simulink model "VARIACION_P5"  (R2019b)
settings: Solver=VariableStepAuto  StartTime=0.0  StopTime=15000  RelTol=1e-3
undefined symbols (not defined in the file): n, p1, p2, p3, p6
libraries: simulink x10
settings Model: Creator=USUARIO  LastModifiedBy=USUARIO

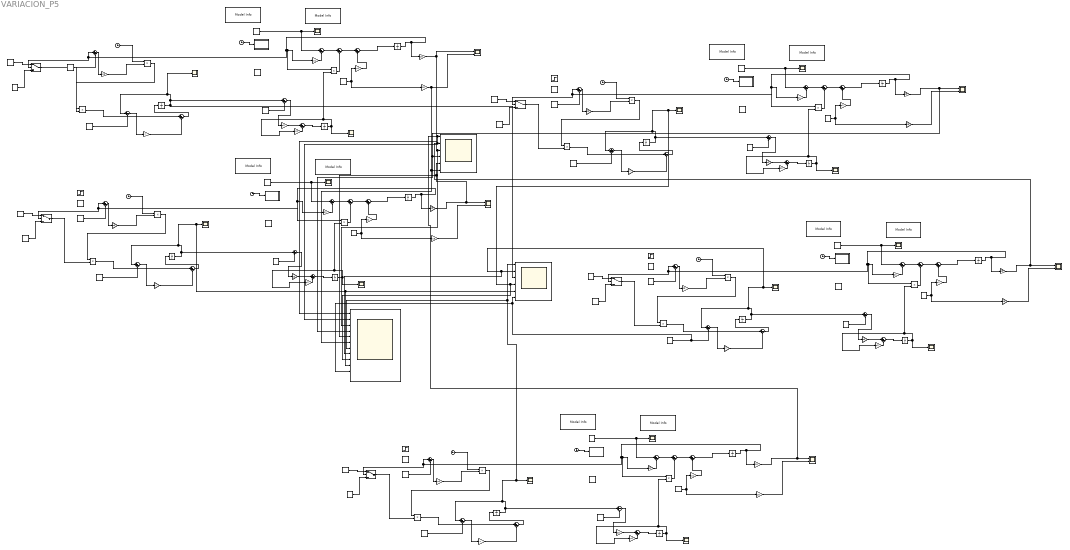
== system VARIACION_P5 ==
  Clock{,1..9} (10 alike) : Clock
  Constant{1..5} (5 alike) : Constant  Value=0
  Gain{1,5,7,11,13,17,19,23,25,29} (10 alike) : Gain  Gain=p1
  Gain{3..4,9..10,15..16,21..22,27..28} (10 alike) : Gain  Gain=18
  Gain{6,12,18,24,30} (5 alike) : Gain  Gain=p2
  Gain{2,8,14,20,26} (5 alike) : Gain  Gain=p3
  Glucosa {,1..3} (4 alike) : Constant  Value=7
  Glucosa basal{1..2,5,10,13} (5 alike) : Constant  Value=4.5
  Glucosa basal{3,6..7,11,14} (5 alike) : Constant
  Glucosa basal{4,8..9,12,15} (5 alike) : Constant  Value=0
  Grafica ingesta D{1..5} (5 alike) : Scope
  INSULINA{,1..4} (5 alike) : Scope
  Ib{,1..4} (5 alike) : Constant  Value=12
  Ingesta 75 g1 : MATLAB Function  TreatAsAtomicUnit=on
  Ingesta 75 g2 : MATLAB Function  TreatAsAtomicUnit=on
  Ingesta 75 g3 : MATLAB Function  TreatAsAtomicUnit=on
  Ingesta 75 g4 : MATLAB Function  TreatAsAtomicUnit=on
  Ingesta 75 g5 : MATLAB Function  TreatAsAtomicUnit=on
  Insulina basal{1..5} (5 alike) : Constant  Value=12
  Integrator{1,3,6,9,15} (5 alike) : Integrator  InitialCondition=7.5
  Integrator{4,7,10,12,14} (5 alike) : Integrator  InitialCondition=12
  Integrator{2,5,8,11,13} (5 alike) : Integrator
  Model Info1 : simulink/Model-Wide Utilities/Model Info  Frame=on  DisplayStringWithTags=|  HorizontalTextAlignment=Center  LeftAlignmentValue=0.5
      | Insulina constante 
      | igual a la basal
      | 
      | I(0) = Ib
  Model Info10 : simulink/Model-Wide Utilities/Model Info  Frame=on  DisplayStringWithTags=|  HorizontalTextAlignment=Center  LeftAlignmentValue=0.5
      | MODELO ORIGINAL
      | 
      | 
      | PERSONA NO DIABETICA
      | 
      | CON INSULINA VARIABLE
  Model Info2 : simulink/Model-Wide Utilities/Model Info  Frame=on  DisplayStringWithTags=|  HorizontalTextAlignment=Center  LeftAlignmentValue=0.5
      | MODELO ORIGINAL
      | 
      | 
      | PERSONA NO DIABETICA
      | 
      | CON INSULINA VARIABLE
  Model Info3 : simulink/Model-Wide Utilities/Model Info  Frame=on  DisplayStringWithTags=|  HorizontalTextAlignment=Center  LeftAlignmentValue=0.5
      | Insulina constante 
      | igual a la basal
      | 
      | I(0) = Ib
  Model Info4 : simulink/Model-Wide Utilities/Model Info  Frame=on  DisplayStringWithTags=|  HorizontalTextAlignment=Center  LeftAlignmentValue=0.5
      | MODELO ORIGINAL
      | 
      | 
      | PERSONA NO DIABETICA
      | 
      | CON INSULINA VARIABLE
  Model Info5 : simulink/Model-Wide Utilities/Model Info  Frame=on  DisplayStringWithTags=|  HorizontalTextAlignment=Center  LeftAlignmentValue=0.5
      | Insulina constante 
      | igual a la basal
      | 
      | I(0) = Ib
  Model Info6 : simulink/Model-Wide Utilities/Model Info  Frame=on  DisplayStringWithTags=|  HorizontalTextAlignment=Center  LeftAlignmentValue=0.5
      | MODELO ORIGINAL
      | 
      | 
      | PERSONA NO DIABETICA
      | 
      | CON INSULINA VARIABLE
  Model Info7 : simulink/Model-Wide Utilities/Model Info  Frame=on  DisplayStringWithTags=|  HorizontalTextAlignment=Center  LeftAlignmentValue=0.5
      | Insulina constante 
      | igual a la basal
      | 
      | I(0) = Ib
  Model Info8 : simulink/Model-Wide Utilities/Model Info  Frame=on  DisplayStringWithTags=|  HorizontalTextAlignment=Center  LeftAlignmentValue=0.5
      | MODELO ORIGINAL
      | 
      | 
      | PERSONA NO DIABETICA
      | 
      | CON INSULINA VARIABLE
  Model Info9 : simulink/Model-Wide Utilities/Model Info  Frame=on  DisplayStringWithTags=|  HorizontalTextAlignment=Center  LeftAlignmentValue=0.5
      | Insulina constante 
      | igual a la basal
      | 
      | I(0) = Ib
  Product{1..15} (15 alike) : Product
  Step{,1..3} (4 alike) : Step  Time=10  Before=7  After=4  SampleTime=0
  Sum{1..2,4..7,9..15,17..23,25..34,36..40} (35 alike) : Sum  Inputs=|+-
  Sum{3,8,16,24,35} (5 alike) : Sum  Inputs=|++
  Switch : Switch  Criteria=u2 > Threshold  Threshold=5
  Switch1 : Switch  Criteria=u2 > Threshold  Threshold=5.556
  Switch2 : Switch  Criteria=u2 > Threshold  Threshold=5.278
  Switch3 : Switch  Criteria=u2 > Threshold  Threshold=4.7222
  Switch4 : Switch  Criteria=u2 > Threshold  Threshold=4.5
  i(T){1..5} (5 alike) : Constant  Value=12
  insulina activa{1..5} (5 alike) : Scope
  mODELO ORIGINAL{1..5} (5 alike) : Scope  NumInputPorts=2
  p1 : Constant  Value=5.56
  p{2,4,6,8,10} (5 alike) : Gain  Gain=p6
  p3 : Constant  Value=5
  p4 = n{,1..4} (5 alike) : Gain  Gain=n
  p5 : Constant  Value=5
  p7 : Constant  Value=5
  p9 : Constant  Value=4.5
  variacion p5: glucosa : Scope  NumInputPorts=6
  variacion p5: glucosa1 : Scope  NumInputPorts=12
  variacion p5: insulina : Scope  NumInputPorts=6
  wires:
  Gain3/1 -> mODELO ORIGINAL1/1, variacion p5: glucosa1/3, variacion p5: glucosa/3  "Caso base: glucosa para p5 = 90 mg/dL"
  Sum33/1 -> Integrator14/1
  Glucosa basal7/1 -> Switch/1  "glucosa basal"
  Sum4/1 -> Integrator2/1
  Clock1/1 -> Ingesta 75 g1/1(in)
  Product7/1 -> Product8/1
  Glucosa basal1/1 -> Gain5/1, Gain4/1  "glucosa basal"
  Integrator1/1 -> Gain3/1, Sum31/1, Switch/2, Product1/1, Gain1/1  "G(t)"
  Gain2/1 -> Sum4/1
  Sum1/1 -> Gain2/1
  p5/1 -> Sum31/2  "glucosa basal"
  Sum5/1 -> Sum3/1
  Insulina basal1/1 -> Sum1/2  "insulina basal"
  Gain1/1 -> Sum2/2
  Ib/1 -> Sum32/2  "glucosa basal"
  Gain6/1 -> Sum4/2
  Sum2/1 -> Sum5/1
  Product1/1 -> Sum5/2
  Constant1/1 -> Grafica ingesta D1/1, Sum2/1
  Gain5/1 -> Sum3/2
  Sum32/1 -> p4 = n/1
  Switch/1 -> Product8/2
  Clock/1 -> Product7/1
  Glucosa basal8/1 -> Switch/3  "glucosa basal"
  Integrator14/1 -> variacion p5: insulina/3, INSULINA/1, Sum32/1, Sum1/1  "Caso base: insulina para p5=90 mg/dL"
  Gain4/1 -> variacion p5: glucosa/6, variacion p5: glucosa1/6, mODELO ORIGINAL1/2  "glucosa basal"
  Sum3/1 -> Integrator1/1
  Sum31/1 -> p6/1
  Product8/1 -> Sum33/1
  Integrator2/1 -> insulina activa1/1, Product1/2, Gain6/1  "X(t)"
  p4 = n/1 -> Sum33/2
  p6/1 -> Product7/2
  Gain9/1 -> variacion p5: glucosa/5, variacion p5: glucosa1/5, mODELO ORIGINAL2/1  "Glucosa para p5 = 100 mg/dL"
  Sum11/1 -> Integrator4/1
  Glucosa basal3/1 -> Switch1/1  "glucosa basal"
  Sum12/1 -> Integrator5/1
  Clock3/1 -> Ingesta 75 g2/1(in)
  Product3/1 -> Product4/1
  Glucosa basal2/1 -> Gain11/1, Gain10/1  "glucosa basal"
  Integrator3/1 -> Gain9/1, Sum9/1, Switch1/2, Product2/1, Gain7/1  "G(t)"
  Gain8/1 -> Sum12/1
  Sum6/1 -> Gain8/1
  p1/1 -> Sum9/2  "glucosa basal"
  Sum13/1 -> Sum8/1
  Insulina basal2/1 -> Sum6/2  "insulina basal"
  Gain7/1 -> Sum7/2
  Ib1/1 -> Sum10/2  "glucosa basal"
  Gain12/1 -> Sum12/2
  Sum7/1 -> Sum13/1
  Product2/1 -> Sum13/2
  Constant2/1 -> Grafica ingesta D2/1, Sum7/1
  Gain11/1 -> Sum8/2
  Sum10/1 -> p4 = n1/1
  Switch1/1 -> Product4/2
  Clock2/1 -> Product3/1
  Glucosa basal4/1 -> Switch1/3  "glucosa basal"
  Integrator4/1 -> Sum6/1, variacion p5: insulina/5, variacion p5: glucosa1/10, INSULINA1/1, Sum10/1  "Insulina para p5 = 100 mg/dL"
  Gain10/1 -> mODELO ORIGINAL2/2  "glucosa basal"
  Sum8/1 -> Integrator3/1
  Sum9/1 -> p2/1
  Product4/1 -> Sum11/1
  Integrator5/1 -> insulina activa2/1, Product2/2, Gain12/1  "X(t)"
  p4 = n1/1 -> Sum11/2
  p2/1 -> Product3/2
  Gain15/1 -> variacion p5: glucosa/4, variacion p5: glucosa1/4, mODELO ORIGINAL3/1  "Glucosa para p5 = 95 mg/dL"
  Sum19/1 -> Integrator7/1
  Glucosa basal6/1 -> Switch2/1  "glucosa basal"
  Sum20/1 -> Integrator8/1
  Clock5/1 -> Ingesta 75 g3/1(in)
  Product6/1 -> Product9/1
  Glucosa basal5/1 -> Gain17/1, Gain16/1  "glucosa basal"
  Integrator6/1 -> Gain15/1, Sum17/1, Switch2/2, Product5/1, Gain13/1  "G(t)"
  Gain14/1 -> Sum20/1
  Sum14/1 -> Gain14/1
  p3/1 -> Sum17/2  "glucosa basal"
  Sum21/1 -> Sum16/1
  Insulina basal3/1 -> Sum14/2  "insulina basal"
  Gain13/1 -> Sum15/2
  Ib2/1 -> Sum18/2  "glucosa basal"
  Gain18/1 -> Sum20/2
  Sum15/1 -> Sum21/1
  Product5/1 -> Sum21/2
  Constant3/1 -> Grafica ingesta D3/1, Sum15/1
  Gain17/1 -> Sum16/2
  Sum18/1 -> p4 = n2/1
  Switch2/1 -> Product9/2
  Clock4/1 -> Product6/1
  Glucosa basal9/1 -> Switch2/3  "glucosa basal"
  Integrator7/1 -> Sum14/1, variacion p5: glucosa1/9, variacion p5: insulina/4, INSULINA2/1, Sum18/1  "Insulina para p5 = 95 mg/dL"
  Gain16/1 -> mODELO ORIGINAL3/2  "glucosa basal"
  Sum16/1 -> Integrator6/1
  Sum17/1 -> p4/1
  Product9/1 -> Sum19/1
  Integrator8/1 -> insulina activa3/1, Product5/2, Gain18/1  "X(t)"
  p4 = n2/1 -> Sum19/2
  p4/1 -> Product6/2
  Gain21/1 -> variacion p5: glucosa1/2, variacion p5: glucosa/2, mODELO ORIGINAL4/1  "Glucosa para p5 = 85 mg/dL"
  Sum27/1 -> Integrator10/1
  Glucosa basal11/1 -> Switch3/1  "glucosa basal"
  Sum28/1 -> Integrator11/1
  Clock7/1 -> Ingesta 75 g4/1(in)
  Product11/1 -> Product12/1
  Glucosa basal10/1 -> Gain23/1, Gain22/1  "glucosa basal"
  Integrator9/1 -> Gain21/1, Sum25/1, Switch3/2, Product10/1, Gain19/1  "G(t)"
  Gain20/1 -> Sum28/1
  Sum22/1 -> Gain20/1
  p7/1 -> Sum25/2  "glucosa basal"
  Sum29/1 -> Sum24/1
  Insulina basal4/1 -> Sum22/2  "insulina basal"
  Gain19/1 -> Sum23/2
  Ib3/1 -> variacion p5: glucosa1/11, variacion p5: insulina/6, Sum26/2  "insulina basal"
  Gain24/1 -> Sum28/2
  Sum23/1 -> Sum29/1
  Product10/1 -> Sum29/2
  Constant4/1 -> Grafica ingesta D4/1, Sum23/1
  Gain23/1 -> Sum24/2
  Sum26/1 -> p4 = n3/1
  Switch3/1 -> Product12/2
  Clock6/1 -> Product11/1
  Glucosa basal12/1 -> Switch3/3  "glucosa basal"
  Integrator10/1 -> Sum22/1, variacion p5: glucosa1/8, variacion p5: insulina/2, INSULINA3/1, Sum26/1  "Insulina para p5 = 85 mg/dL"
  Gain22/1 -> mODELO ORIGINAL4/2  "glucosa basal"
  Sum24/1 -> Integrator9/1
  Sum25/1 -> p8/1
  Product12/1 -> Sum27/1
  Integrator11/1 -> insulina activa4/1, Product10/2, Gain24/1  "X(t)"
  p4 = n3/1 -> Sum27/2
  p8/1 -> Product11/2
  Integrator13/1 -> insulina activa5/1, Product13/2, Gain30/1  "X(t)"
  Sum36/1 -> p10/1
  Sum35/1 -> Integrator15/1
  Product15/1 -> Sum38/1
  Gain28/1 -> mODELO ORIGINAL5/2  "glucosa basal"
  Integrator12/1 -> Sum30/1, variacion p5: insulina/1, variacion p5: glucosa1/7, INSULINA4/1, Sum37/1  "Insulina para p5 = 81 mg/dL= Gb"
  Sum37/1 -> p4 = n4/1
  Clock8/1 -> Product14/1
  Sum40/1 -> Sum35/1
  Gain30/1 -> Sum39/2
  Switch4/1 -> Product15/2
  Sum34/1 -> Sum40/1
  Gain29/1 -> Sum35/2
  Ib4/1 -> Sum37/2  "glucosa basal"
  Insulina basal5/1 -> Sum30/2  "insulina basal"
  Product13/1 -> Sum40/2
  p9/1 -> Sum36/2  "glucosa basal"
  p10/1 -> Product14/2
  Integrator15/1 -> Gain27/1, Sum36/1, Switch4/2, Product13/1, Gain25/1  "G(t)"
  Gain25/1 -> Sum34/2
  Gain26/1 -> Sum39/1
  Sum39/1 -> Integrator13/1
  Glucosa basal15/1 -> Switch4/3  "glucosa basal"
  Product14/1 -> Product15/1
  Sum30/1 -> Gain26/1
  Glucosa basal13/1 -> Gain29/1, Gain28/1  "glucosa basal"
  Constant5/1 -> Grafica ingesta D5/1, Sum34/1
  Sum38/1 -> Integrator12/1
  Glucosa basal14/1 -> Switch4/1  "glucosa basal"
  Gain27/1 -> variacion p5: glucosa1/1, variacion p5: glucosa/1, mODELO ORIGINAL5/1  "Glucosa para p5 = 81 mg/dL= Gb"
  Clock9/1 -> Ingesta 75 g5/1(in)
  p4 = n4/1 -> Sum38/2

== matlab function VARIACION_P5/Ingesta 75 g1 ==
  data: in input; D output
function D = comida(in)
% Variables de entrada en la funcion
t = in(1) %- 8*60*60; % Ajuste para iniciar a las 8 de la mañana
 
% Parámetros del modelo
Ag = 0.8; % adimensional
Tmaxi = 55*60; % s
Vg = 13.79; % L
Tmaxg = 40*60; % s
t1 = 0;
Dg = 0;
f = 1000/180; % factor de conversión de g a mmol
 
% Comidas (perturbaciones) a lo largo de un día
if t >= 0 && t < 180*60 % ingesta de 75 g de HC
    t1 = 0;
    Dg = 50*f;
end
 
% Ecuación
D = (Dg*Ag*(t-t1)*exp(-(t-t1)/Tmaxi))/(Vg*Tmaxg^2);

== matlab function VARIACION_P5/Ingesta 75 g2 ==
  data: in input; D output
function D = comida(in)
% Variables de entrada en la funcion
t = in(1) %- 8*60*60; % Ajuste para iniciar a las 8 de la mañana
 
% Parámetros del modelo
Ag = 0.8; % adimensional
Tmaxi = 55*60; % s
Vg = 13.79; % L
Tmaxg = 40*60; % s
t1 = 0;
Dg = 0;
f = 1000/180; % factor de conversión de g a mmol
 
% Comidas (perturbaciones) a lo largo de un día
if t >= 0 && t < 180*60 % ingesta de 75 g de HC
    t1 = 0;
    Dg = 50*f;
end
 
% Ecuación
D = (Dg*Ag*(t-t1)*exp(-(t-t1)/Tmaxi))/(Vg*Tmaxg^2);

== matlab function VARIACION_P5/Ingesta 75 g3 ==
  data: in input; D output
function D = comida(in)
% Variables de entrada en la funcion
t = in(1) %- 8*60*60; % Ajuste para iniciar a las 8 de la mañana
 
% Parámetros del modelo
Ag = 0.8; % adimensional
Tmaxi = 55*60; % s
Vg = 13.79; % L
Tmaxg = 40*60; % s
t1 = 0;
Dg = 0;
f = 1000/180; % factor de conversión de g a mmol
 
% Comidas (perturbaciones) a lo largo de un día
if t >= 0 && t < 180*60 % ingesta de 75 g de HC
    t1 = 0;
    Dg = 50*f;
end
 
% Ecuación
D = (Dg*Ag*(t-t1)*exp(-(t-t1)/Tmaxi))/(Vg*Tmaxg^2);

== matlab function VARIACION_P5/Ingesta 75 g4 ==
  data: in input; D output
function D = comida(in)
% Variables de entrada en la funcion
t = in(1) %- 8*60*60; % Ajuste para iniciar a las 8 de la mañana
 
% Parámetros del modelo
Ag = 0.8; % adimensional
Tmaxi = 55*60; % s
Vg = 13.79; % L
Tmaxg = 40*60; % s
t1 = 0;
Dg = 0;
f = 1000/180; % factor de conversión de g a mmol
 
% Comidas (perturbaciones) a lo largo de un día
if t >= 0 && t < 180*60 % ingesta de 75 g de HC
    t1 = 0;
    Dg = 50*f;
end
 
% Ecuación
D = (Dg*Ag*(t-t1)*exp(-(t-t1)/Tmaxi))/(Vg*Tmaxg^2);

== matlab function VARIACION_P5/Ingesta 75 g5 ==
  data: in input; D output
function D = comida(in)
% Variables de entrada en la funcion
t = in(1) %- 8*60*60; % Ajuste para iniciar a las 8 de la mañana
 
% Parámetros del modelo
Ag = 0.8; % adimensional
Tmaxi = 55*60; % s
Vg = 13.79; % L
Tmaxg = 40*60; % s
t1 = 0;
Dg = 0;
f = 1000/180; % factor de conversión de g a mmol
 
% Comidas (perturbaciones) a lo largo de un día
if t >= 0 && t < 180*60 % ingesta de 75 g de HC
    t1 = 0;
    Dg = 50*f;
end
 
% Ecuación
D = (Dg*Ag*(t-t1)*exp(-(t-t1)/Tmaxi))/(Vg*Tmaxg^2);
